simulink model "PendulumRCSPlant"  (R2018b)
settings: Solver=VariableStepAuto  StartTime=0.0  StopTime=20  RelTol=1e-9
values from neighbouring files (symbols this model uses):
  Delayx = 1    [LinearizePendulumRCSPlant.m]    (also in TestFullStateFeedback.m = Delay(1, i); TestPendulumRCSPlant.m = Delay(1, i); TestPendulumRCSPlantWPsi.m = Delay(1, i); TestQuantizedFullStateFeedback.m = Delay(1, i))
  Delayy = 1    [LinearizePendulumRCSPlant.m]    (also in TestFullStateFeedback.m = Delay(2, i); TestPendulumRCSPlant.m = Delay(2, i); TestPendulumRCSPlantWPsi.m = Delay(2, i); TestQuantizedFullStateFeedback.m = Delay(2, i))
  Fx = 0    [LinearizePendulumRCSPlant.m]    (also in TestFullStateFeedback.m = Fe(1, i); TestPendulumRCSPlant.m = Fe(1, i); TestPendulumRCSPlantWPsi.m = Fe(1, i); TestQuantizedFullStateFeedback.m = Fe(1, i))
  Fy = 0    [LinearizePendulumRCSPlant.m]    (also in TestFullStateFeedback.m = Fe(2, i); TestPendulumRCSPlant.m = Fe(2, i); TestPendulumRCSPlantWPsi.m = Fe(2, i); TestQuantizedFullStateFeedback.m = Fe(2, i))
  L = 3    [GenPendulumParams.m]
  M = 1.79    [GenPendulumParams.m]
libraries: sharedutil x1, shared6dof x1, aerolibanim x1, vrlib x1
settings Model: OrderedModelArguments=off  Creator=mendicantbias  LastModifiedBy=mendicantbias
settings ModelReferenceCC: ModelReferenceNumInstancesAllowed=Single

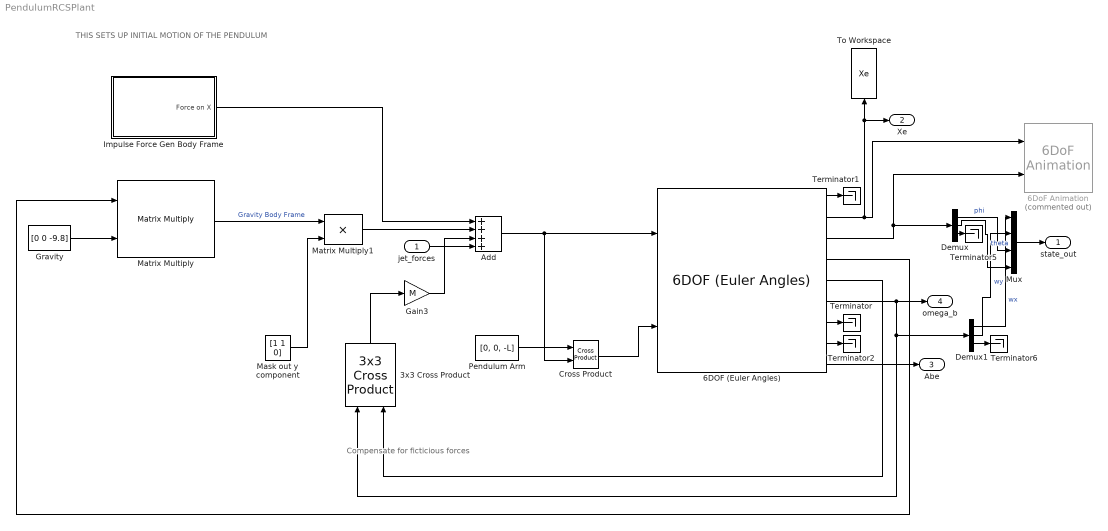
== system PendulumRCSPlant ==
  note: THIS SETS UP INITIAL MOTION OF THE PENDULUM
  note: Compensate for ficticious forces
  jet_forces : Inport  PortDimensions=3
  3x3 Cross Product : sharedutil/3x3 Cross Product  aMode=aMode
      settings: SourceProductBaseCode=AE
  6DOF (Euler Angles) : shared6dof/6DOF (Euler Angles)  units=Metric (MKS)  mtype=Fixed  rep=Euler Angles  xme_0=[0 0 -L]  Vm_0=[0 0 0]  eul_0=[0 0 0]  pm_0=[0 0 0]  mass_0=M  mass_e=0.5  mass_f=2.0  inertia=I  inertia_e=eye(3)  inertia_f=2*eye(3)  k_quat=1.0  vre_flag=on  abi_flag=on  aMode=0  xme_statename=''  Vm_statename=''  eul_statename=''  quat_statename=''  pm_statename=''  mass_statename=''
      settings: SourceProductBaseCode=AE
  6DoF Animation : aerolibanim/6DoF Animation  Commented=on  u1=[-10, 10, -10, 10, -10, 10]  u2=0.1  u3=0.5  u4=[0 0 0]  u5=Fixed position  u6=[3 3 3]  u7=30  u8=on
      settings: SourceProductName=Aerospace Blockset
  Add : Sum  Inputs=++++
  Cross Product : vrlib/Utilities/Cross Product
      settings: SourceProductBaseCode=VR
  Demux : Demux  Outputs=3
  Demux1 : Demux  Outputs=3
  Gain3 : Gain  Gain=M
  Gravity : Constant  Value=[0 0 -9.8]
  Impulse Force Gen Body Frame : Subsystem
  Mask out y component : Constant  Value=[1 1 0]
  Matrix Multiply : Product  Multiplication=Matrix(*)
  Matrix Multiply1 : Product
  Mux : Mux
  Pendulum Arm : Constant  Value=[0, 0, -L]
  Terminator{,1..2,5..6} (5 alike) : Terminator
  To Workspace : ToWorkspace  VariableName=Xe  SaveFormat=Timeseries  SampleTime=-1
  state_out : Outport
  Xe : Outport  Port=2
  Abe : Outport  Port=3
  omega_b : Outport  Port=4
  wires:
  Matrix Multiply/1 -> Matrix Multiply1/1  "Gravity Body Frame"
  Gravity/1 -> Matrix Multiply/2
  6DOF (Euler Angles)/4 -> Matrix Multiply/1
  Add/1 -> 6DOF (Euler Angles)/1, Cross Product/2
  Pendulum Arm/1 -> Cross Product/1
  Cross Product/1 -> 6DOF (Euler Angles)/2
  6DOF (Euler Angles)/6 -> omega_b/1, Demux1/1, 3x3 Cross Product/1
  6DOF (Euler Angles)/5 -> 3x3 Cross Product/2
  Mask out y component/1 -> Matrix Multiply1/2
  Matrix Multiply1/1 -> Add/2
  Impulse Force Gen Body Frame/1(Force on X) -> Add/1
  3x3 Cross Product/1 -> Gain3/1
  Gain3/1 -> Add/3
  6DOF (Euler Angles)/7 -> Terminator/1
  6DOF (Euler Angles)/1 -> Terminator1/1
  6DOF (Euler Angles)/8 -> Terminator2/1
  6DOF (Euler Angles)/2 -> 6DoF Animation/1, To Workspace/1, Xe/1
  6DOF (Euler Angles)/3 -> 6DoF Animation/2, Demux/1
  Demux/3 -> Terminator5/1
  Demux1/3 -> Terminator6/1
  6DOF (Euler Angles)/9 -> Abe/1
  jet_forces/1 -> Add/4
  Mux/1 -> state_out/1
  Demux/1 -> Mux/3  "phi"
  Demux/2 -> Mux/4  "theta"
  Demux1/1 -> Mux/1  "wx"
  Demux1/2 -> Mux/2  "wy"

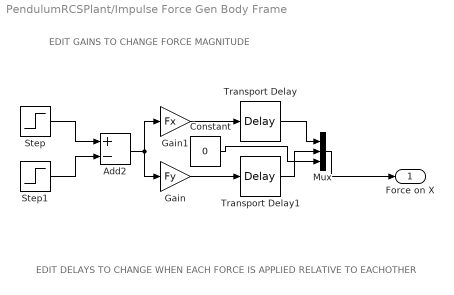
== system PendulumRCSPlant/Impulse Force Gen Body Frame ==
  note: EDIT DELAYS TO CHANGE WHEN EACH FORCE IS APPLIED RELATIVE TO EACHOTHER
  note: EDIT GAINS TO CHANGE FORCE MAGNITUDE
  Add2 : Sum  Inputs=+-
  Constant : Constant  Value=0
  Gain : Gain  Gain=Fy
  Gain1 : Gain  Gain=Fx
  Mux : Mux  Inputs=3
  Step : Step  Time=0  SampleTime=0
  Step1 : Step  SampleTime=0
  Transport Delay : TransportDelay  DelayTime=Delayx
  Transport Delay1 : TransportDelay  DelayTime=Delayy
  Force on X : Outport
  wires:
  Step/1 -> Add2/1
  Step1/1 -> Add2/2
  Add2/1 -> Gain/1, Gain1/1
  Gain1/1 -> Transport Delay/1
  Mux/1 -> Force on X/1
  Gain/1 -> Transport Delay1/1
  Transport Delay/1 -> Mux/1
  Transport Delay1/1 -> Mux/2
  Constant/1 -> Mux/3
